simulink model "sway_simulation"  (R2020a)
settings: Solver=VariableStepAuto  StartTime=0.0  StopTime=10  RelTol=1e-3
values from neighbouring files (symbols this model uses):
  Ag = 1    [swaymotion.m]
  g = 9.8    [swaymotion.m]
  ig1_init = 0    [swaymotion.m]
  ig3_init = 0    [swaymotion.m]
  ig4_init = 0    [swaymotion.m]
  Jz = 2850    [swaymotion.m]
  K = lqr(A,B,Q,Rr)    [swaymotion.m]
  m = 623    [swaymotion.m]
  mu0 = 1.2566*10^(-6)    (= 1.2566e-06)    [swaymotion.m]
  Ng = 10000    [swaymotion.m]
  P1 = 1    [swaymotion.m]
  P2 = 1    [swaymotion.m]
  P3 = 1    [swaymotion.m]
  P4 = 1    [swaymotion.m]
  P5 = 1    [swaymotion.m]
  P6 = 1    [swaymotion.m]
  phi = 0    [swaymotion.m]
  psi_init = 0    [swaymotion.m]
  R = diag([weight_Vg1 weight_Vg2 weight_Vg3 weight_Vg4 weight_Vg5 weight_Vg6])    [swaymotion.m]
  Ra = 0    [swaymotion.m]
  vx = 400/3.6    (= 111.111111111)    [swaymotion.m]
  vy_init = 0    [swaymotion.m]
  wpsi = wpsi_ref    (= 0)    [swaymotion.m]
  wpsi_init = 0    [swaymotion.m]
  x_ref = [y_ref; vy_ref; psi_ref; wpsi_ref; ig_ref; ig_ref; ig_ref; ig_ref; ig_ref; ig_ref]    [swaymotion.m]
  xB = 1    [swaymotion.m]
  y_init = -0.015    [swaymotion.m]
  yB = 1    [swaymotion.m]
  ymax = 0.1    [swaymotion.m]
settings Model: Creator=Federico  LastModifiedBy=Federico

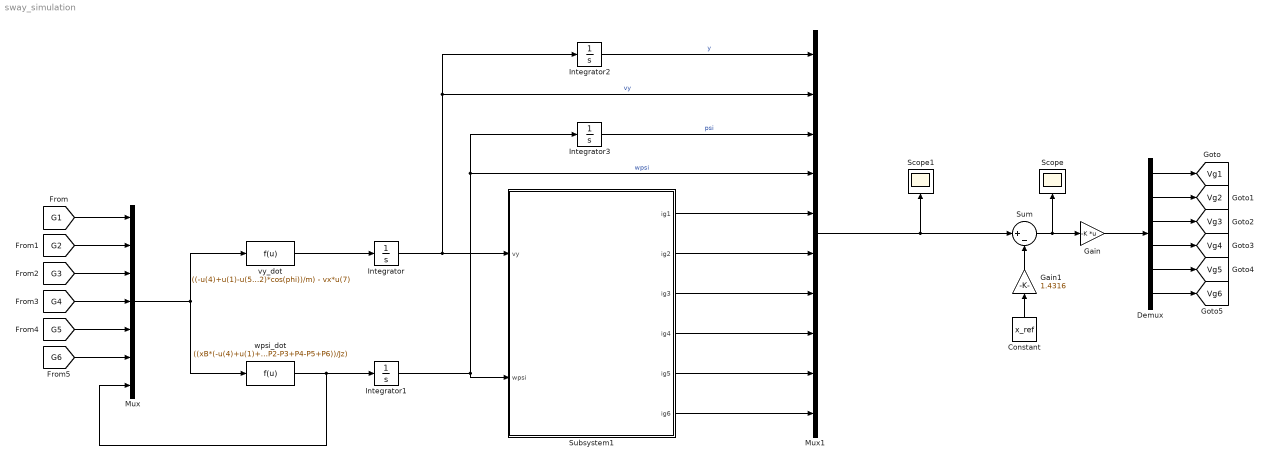
== system sway_simulation ==
  Constant : Constant  Value=x_ref
  Demux : Demux  Outputs=6
  Gain : Gain  Gain=-K  Multiplication=Matrix(K*u)
  Gain1 : Gain  Gain=1.4316
  Integrator : Integrator  InitialCondition=vy_init
  Integrator1 : Integrator  InitialCondition=wpsi_init
  Integrator2 : Integrator  InitialCondition=y_init
  Integrator3 : Integrator  InitialCondition=psi_init
  Mux : Mux  Inputs=7
  Mux1 : Mux  Inputs=10
  Scope : Scope
  Scope1 : Scope
  Subsystem1 : Subsystem
  Sum : Sum  Inputs=|+-
  vy_dot : Fcn  Expr=((-u(4)+u(1)-u(5)+u(2)-u(6)+u(3)+m*g*sin(phi)-m*Ra*(wpsi^2)*cos(phi))/m) - vx*u(7)
  wpsi_dot : Fcn  Expr=((xB*(-u(4)+u(1)+u(6)-u(3))+yB*(-P1+P2-P3+P4-P5+P6))/Jz)
  tag scope: Vg1=global, Vg2=global, Vg3=global, Vg4=global, Vg5=global, Vg6=global
  wires:
  vy_dot/1 -> Integrator/1
  wpsi_dot/1 -> Mux/7, Integrator1/1
  Integrator/1 -> Integrator2/1, Mux1/2, Subsystem1/1(vy)  "vy"
  Integrator1/1 -> Integrator3/1, Mux1/4, Subsystem1/2(wpsi)  "wpsi"
  Mux/1 -> wpsi_dot/1, vy_dot/1
  [G1] -> Mux/1
  [G2] -> Mux/2
  [G3] -> Mux/3
  [G4] -> Mux/4
  [G5] -> Mux/5
  [G6] -> Mux/6
  Integrator2/1 -> Mux1/1  "y"
  Integrator3/1 -> Mux1/3  "psi"
  Subsystem1/1(ig1) -> Mux1/5
  Subsystem1/2(ig2) -> Mux1/6
  Subsystem1/3(ig3) -> Mux1/7
  Subsystem1/4(ig4) -> Mux1/8
  Subsystem1/5(ig5) -> Mux1/9
  Subsystem1/6(ig6) -> Mux1/10
  Gain/1 -> Demux/1
  Demux/1 -> [Vg1]
  Demux/2 -> [Vg2]
  Demux/4 -> [Vg4]
  Demux/3 -> [Vg3]
  Demux/5 -> [Vg5]
  Demux/6 -> [Vg6]
  Mux1/1 -> Scope1/1, Sum/1
  Sum/1 -> Scope/1, Gain/1
  Constant/1 -> Gain1/1
  Gain1/1 -> Sum/2

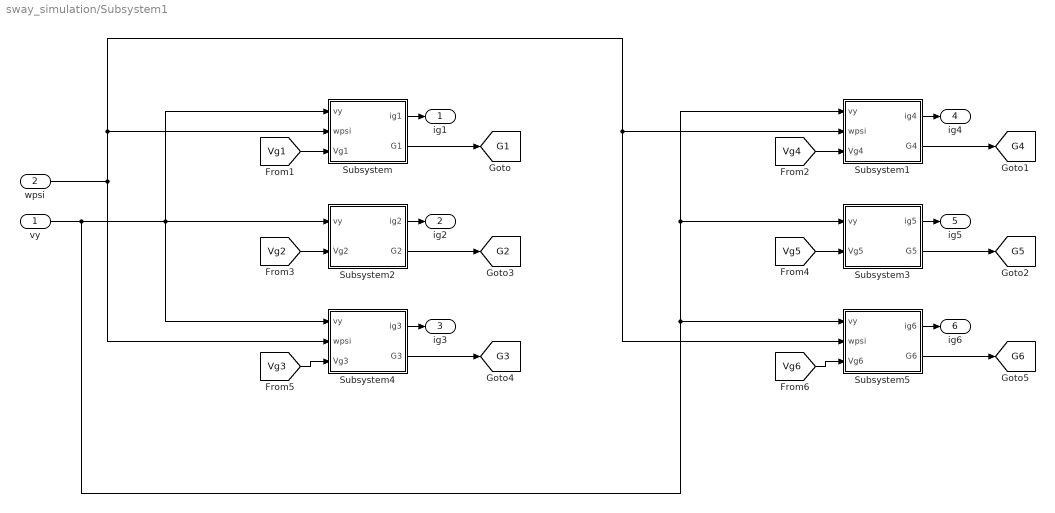
== system sway_simulation/Subsystem1 ==
  vy : Inport
  wpsi : Inport  Port=2
  Subsystem : Subsystem
  Subsystem1 : Subsystem
  Subsystem2 : Subsystem
  Subsystem3 : Subsystem
  Subsystem4 : Subsystem
  Subsystem5 : Subsystem
  ig1 : Outport
  ig2 : Outport  Port=2
  ig3 : Outport  Port=3
  ig4 : Outport  Port=4
  ig5 : Outport  Port=5
  ig6 : Outport  Port=6
  tag scope: G1=global, G2=global, G3=global, G4=global, G5=global, G6=global
  wires:
  Subsystem/2(G1) -> [G1]
  [Vg3] -> Subsystem4/3(Vg3)
  [Vg1] -> Subsystem/3(Vg1)
  Subsystem4/1(ig3) -> ig3/1
  Subsystem/1(ig1) -> ig1/1
  Subsystem2/1(ig2) -> ig2/1
  Subsystem2/2(G2) -> [G2]
  [Vg2] -> Subsystem2/2(Vg2)
  Subsystem4/2(G3) -> [G3]
  Subsystem5/2(G6) -> [G6]
  [Vg5] -> Subsystem3/2(Vg5)
  wpsi/1 -> Subsystem5/2(wpsi), Subsystem1/2(wpsi), Subsystem/2(wpsi), Subsystem4/2(wpsi)
  Subsystem3/2(G5) -> [G5]
  Subsystem3/1(ig5) -> ig5/1
  Subsystem1/1(ig4) -> ig4/1
  Subsystem5/1(ig6) -> ig6/1
  [Vg4] -> Subsystem1/3(Vg4)
  [Vg6] -> Subsystem5/3(Vg6)
  Subsystem1/2(G4) -> [G4]
  vy/1 -> Subsystem2/1(vy), Subsystem/1(vy), Subsystem4/1(vy), Subsystem1/1(vy), Subsystem3/1(vy), Subsystem5/1(vy)

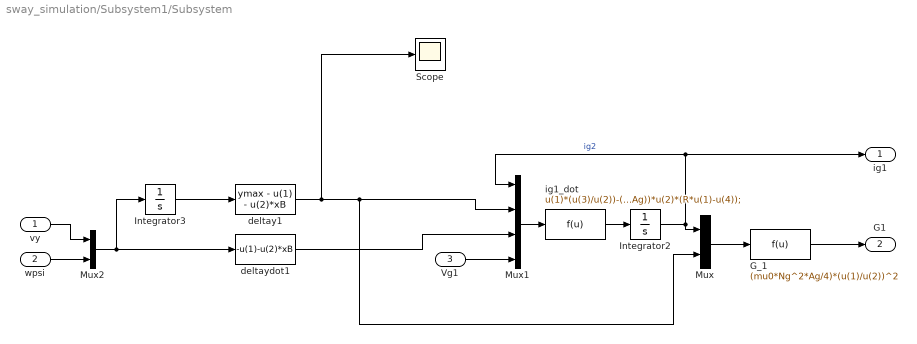
== system sway_simulation/Subsystem1/Subsystem ==
  vy : Inport
  wpsi : Inport  Port=2
  Vg1 : Inport  Port=3
  G_1 : Fcn  Expr=(mu0*Ng^2*Ag/4)*(u(1)/u(2))^2
  Integrator2 : Integrator  InitialCondition=ig1_init
  Integrator3 : Integrator  InitialCondition=[y_init; psi_init]
  Mux : Mux  Inputs=2
  Mux1 : Mux
  Mux2 : Mux  Inputs=2
  Scope : Scope
  deltay1 : Fcn  Expr=ymax - u(1) - u(2)*xB
  deltaydot1 : Fcn  Expr=-u(1)-u(2)*xB
  ig1_dot : Fcn  Expr=u(1)*(u(3)/u(2))-(2/(mu0*(Ng^2)*Ag))*u(2)*(R*u(1)-u(4));
  ig1 : Outport
  G1 : Outport  Port=2
  wires:
  ig1_dot/1 -> Integrator2/1
  G_1/1 -> G1/1
  deltaydot1/1 -> Mux1/3
  vy/1 -> Mux2/1
  Mux2/1 -> Integrator3/1, deltaydot1/1
  Vg1/1 -> Mux1/4
  Mux/1 -> G_1/1
  Integrator2/1 -> Mux/1, ig1/1, Mux1/1  "ig2"
  wpsi/1 -> Mux2/2
  Mux1/1 -> ig1_dot/1
  Integrator3/1 -> deltay1/1
  deltay1/1 -> Scope/1, Mux/2, Mux1/2

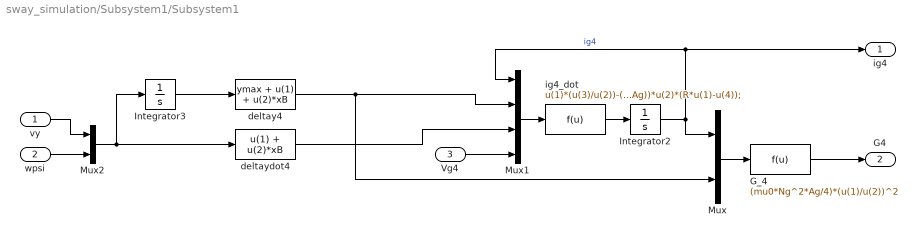
== system sway_simulation/Subsystem1/Subsystem1 ==
  vy : Inport
  wpsi : Inport  Port=2
  Vg4 : Inport  Port=3
  G_4 : Fcn  Expr=(mu0*Ng^2*Ag/4)*(u(1)/u(2))^2
  Integrator2 : Integrator  InitialCondition=ig1_init
  Integrator3 : Integrator  InitialCondition=[y_init; psi_init]
  Mux : Mux  Inputs=2
  Mux1 : Mux
  Mux2 : Mux  Inputs=2
  deltay4 : Fcn  Expr=ymax + u(1) + u(2)*xB
  deltaydot4 : Fcn  Expr=u(1) + u(2)*xB
  ig4_dot : Fcn  Expr=u(1)*(u(3)/u(2))-(2/(mu0*(Ng^2)*Ag))*u(2)*(R*u(1)-u(4));
  ig4 : Outport
  G4 : Outport  Port=2
  wires:
  deltay4/1 -> Mux/2, Mux1/2
  Integrator3/1 -> deltay4/1
  Mux1/1 -> ig4_dot/1
  wpsi/1 -> Mux2/2
  Integrator2/1 -> Mux1/1, ig4/1, Mux/1  "ig4"
  Mux/1 -> G_4/1
  Vg4/1 -> Mux1/4
  Mux2/1 -> deltaydot4/1, Integrator3/1
  vy/1 -> Mux2/1
  deltaydot4/1 -> Mux1/3
  G_4/1 -> G4/1
  ig4_dot/1 -> Integrator2/1

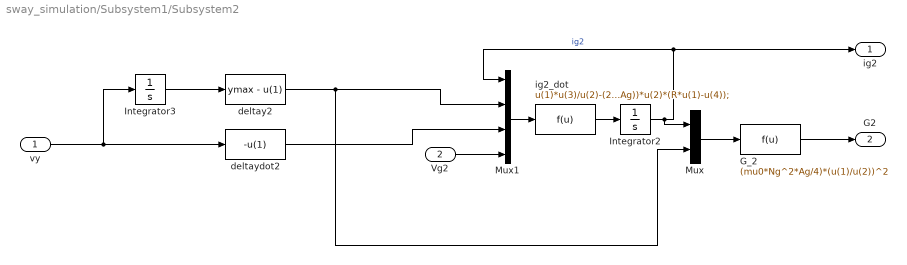
== system sway_simulation/Subsystem1/Subsystem2 ==
  vy : Inport
  Vg2 : Inport  Port=2
  G_2 : Fcn  Expr=(mu0*Ng^2*Ag/4)*(u(1)/u(2))^2
  Integrator2 : Integrator  InitialCondition=ig4_init
  Integrator3 : Integrator  InitialCondition=y_init
  Mux : Mux  Inputs=2
  Mux1 : Mux
  deltay2 : Fcn  Expr=ymax - u(1)
  deltaydot2 : Fcn  Expr=-u(1)
  ig2_dot : Fcn  Expr=u(1)*u(3)/u(2)-(2/(mu0*(Ng^2)*Ag))*u(2)*(R*u(1)-u(4));
  ig2 : Outport
  G2 : Outport  Port=2
  wires:
  deltay2/1 -> Mux/2, Mux1/2
  Integrator3/1 -> deltay2/1
  Mux1/1 -> ig2_dot/1
  Integrator2/1 -> Mux/1, Mux1/1, ig2/1  "ig2"
  Mux/1 -> G_2/1
  Vg2/1 -> Mux1/4
  deltaydot2/1 -> Mux1/3
  G_2/1 -> G2/1
  ig2_dot/1 -> Integrator2/1
  vy/1 -> Integrator3/1, deltaydot2/1

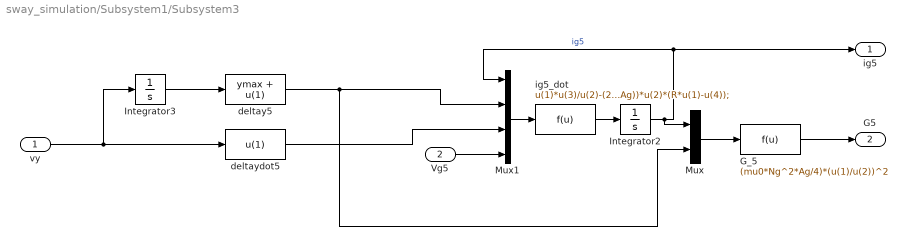
== system sway_simulation/Subsystem1/Subsystem3 ==
  vy : Inport
  Vg5 : Inport  Port=2
  G_5 : Fcn  Expr=(mu0*Ng^2*Ag/4)*(u(1)/u(2))^2
  Integrator2 : Integrator  InitialCondition=ig4_init
  Integrator3 : Integrator  InitialCondition=y_init
  Mux : Mux  Inputs=2
  Mux1 : Mux
  deltay5 : Fcn  Expr=ymax + u(1)
  deltaydot5 : Fcn  Expr=u(1)
  ig5_dot : Fcn  Expr=u(1)*u(3)/u(2)-(2/(mu0*(Ng^2)*Ag))*u(2)*(R*u(1)-u(4));
  ig5 : Outport
  G5 : Outport  Port=2
  wires:
  vy/1 -> deltaydot5/1, Integrator3/1
  ig5_dot/1 -> Integrator2/1
  G_5/1 -> G5/1
  deltaydot5/1 -> Mux1/3
  Vg5/1 -> Mux1/4
  Mux/1 -> G_5/1
  Integrator2/1 -> ig5/1, Mux1/1, Mux/1  "ig5"
  Mux1/1 -> ig5_dot/1
  Integrator3/1 -> deltay5/1
  deltay5/1 -> Mux/2, Mux1/2

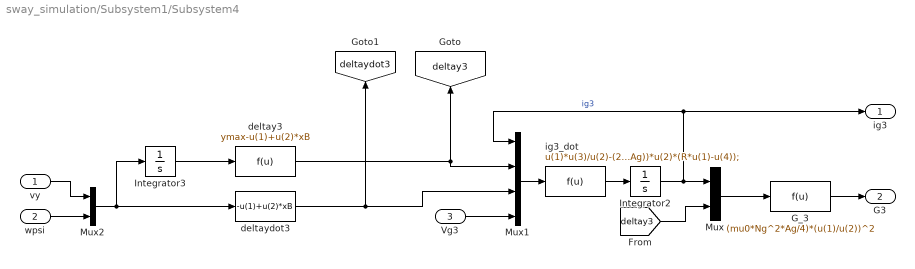
== system sway_simulation/Subsystem1/Subsystem4 ==
  vy : Inport
  wpsi : Inport  Port=2
  Vg3 : Inport  Port=3
  G_3 : Fcn  Expr=(mu0*Ng^2*Ag/4)*(u(1)/u(2))^2
  Integrator2 : Integrator  InitialCondition=ig3_init
  Integrator3 : Integrator  InitialCondition=[y_init; psi_init]
  Mux : Mux  Inputs=2
  Mux1 : Mux
  Mux2 : Mux  Inputs=2
  deltay3 : Fcn  Expr=ymax-u(1)+u(2)*xB
  deltaydot3 : Fcn  Expr=-u(1)+u(2)*xB
  ig3_dot : Fcn  Expr=u(1)*u(3)/u(2)-(2/(mu0*(Ng^2)*Ag))*u(2)*(R*u(1)-u(4));
  ig3 : Outport
  G3 : Outport  Port=2
  tag scope: deltay3=global, deltaydot3=global
  wires:
  ig3_dot/1 -> Integrator2/1
  G_3/1 -> G3/1
  deltaydot3/1 -> Mux1/3, [deltaydot3]
  vy/1 -> Mux2/1
  Mux2/1 -> Integrator3/1, deltaydot3/1
  Vg3/1 -> Mux1/4
  Mux/1 -> G_3/1
  Integrator2/1 -> ig3/1, Mux1/1, Mux/1  "ig3"
  wpsi/1 -> Mux2/2
  [deltay3] -> Mux/2
  Mux1/1 -> ig3_dot/1
  Integrator3/1 -> deltay3/1
  deltay3/1 -> Mux1/2, [deltay3]

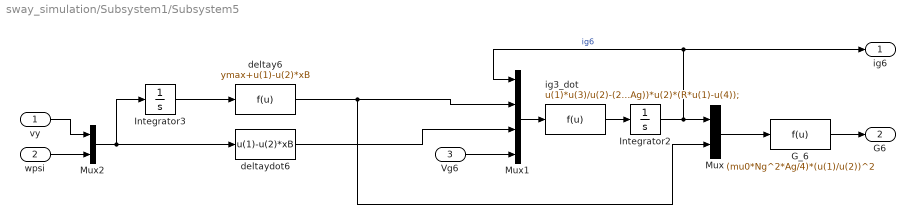
== system sway_simulation/Subsystem1/Subsystem5 ==
  vy : Inport
  wpsi : Inport  Port=2
  Vg6 : Inport  Port=3
  G_6 : Fcn  Expr=(mu0*Ng^2*Ag/4)*(u(1)/u(2))^2
  Integrator2 : Integrator  InitialCondition=ig3_init
  Integrator3 : Integrator  InitialCondition=[y_init; psi_init]
  Mux : Mux  Inputs=2
  Mux1 : Mux
  Mux2 : Mux  Inputs=2
  deltay6 : Fcn  Expr=ymax+u(1)-u(2)*xB
  deltaydot6 : Fcn  Expr=u(1)-u(2)*xB
  ig3_dot : Fcn  Expr=u(1)*u(3)/u(2)-(2/(mu0*(Ng^2)*Ag))*u(2)*(R*u(1)-u(4));
  ig6 : Outport
  G6 : Outport  Port=2
  wires:
  deltay6/1 -> Mux/2, Mux1/2
  Integrator3/1 -> deltay6/1
  Mux1/1 -> ig3_dot/1
  wpsi/1 -> Mux2/2
  Integrator2/1 -> Mux/1, Mux1/1, ig6/1  "ig6"
  Mux/1 -> G_6/1
  Vg6/1 -> Mux1/4
  Mux2/1 -> deltaydot6/1, Integrator3/1
  vy/1 -> Mux2/1
  deltaydot6/1 -> Mux1/3
  G_6/1 -> G6/1
  ig3_dot/1 -> Integrator2/1
